simulink model "pitch_kalman_bias_sim"  (R2021b)
settings: Solver=VariableStepAuto  StartTime=0.0  StopTime=10.0  RelTol=1e-3
values from neighbouring files (symbols this model uses):
  A = [0 w_0(3) -w_0(2) 0 x_0(3) -x_0(2) ... (first row only)    [kalman_ex_5.m]    (also in pitch_kalman.m = 0; pitch_kalman_bias.m = [0 -1;0 0]; roll_kalman.m = 0; roll_kalman_bias.m = [0 -1;0 0])
  B = 1    [pitch_kalman.m]    (also in pitch_kalman_bias.m = [1;0]; roll_kalman.m; roll_kalman_bias.m = [1;0])
  bias = -0.3*ones(3,1)    [kalman_ex_5.m]    (also in pitch_kalman_bias.m = -0.3; roll_kalman_bias.m = -0.3)
  C = [eye(3) zeros(3,3)]    [kalman_ex_5.m]    (also in pitch_kalman.m = 1; pitch_kalman_bias.m = [1 0]; roll_kalman.m = 1; roll_kalman_bias.m = [1 0])
undefined symbols (not defined in the file or in its folder): L
settings Model: Creator=p28ma  LastModifiedBy=p28ma

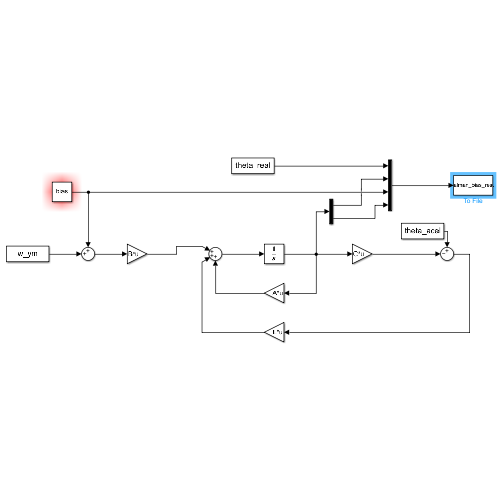
[thumbnail: Simulink's stored preview of the top-level diagram]
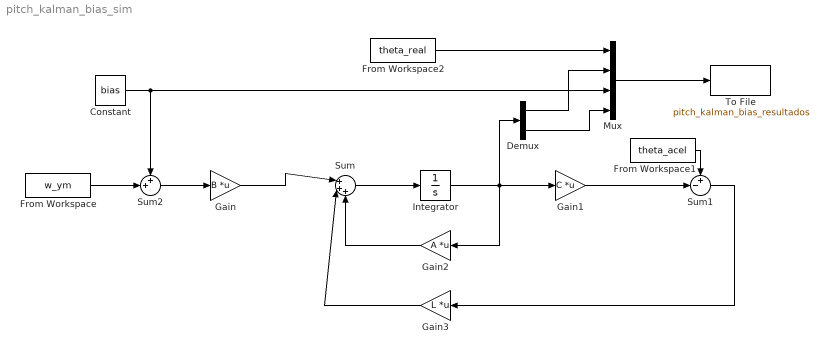
== system pitch_kalman_bias_sim ==
  Constant : Constant  Value=bias
  Demux : Demux  Outputs=2
  From Workspace : FromWorkspace  VariableName=w_ym  OutputAfterFinalValue=Setting to zero
  From Workspace1 : FromWorkspace  VariableName=theta_acel
  From Workspace2 : FromWorkspace  VariableName=theta_real
  Gain : Gain  Gain=B  Multiplication=Matrix(K*u)
  Gain1 : Gain  Gain=C  Multiplication=Matrix(K*u)
  Gain2 : Gain  Gain=A  Multiplication=Matrix(K*u)
  Gain3 : Gain  Gain=L  Multiplication=Matrix(K*u)
  Integrator : Integrator
  Mux : Mux
  Sum : Sum  Inputs=|+++
  Sum1 : Sum  Inputs=+-|
  Sum2 : Sum  Inputs=++|
  To File : ToFile  Filename=pitch_kalman_bias_resultados  MatrixName=pitch_kalman_bias_resultados  SaveFormat=Timeseries
  wires:
  Gain/1 -> Sum/1
  Sum/1 -> Integrator/1
  Integrator/1 -> Demux/1, Gain2/1, Gain1/1
  Gain2/1 -> Sum/3
  Sum1/1 -> Gain3/1
  Gain3/1 -> Sum/2
  Gain1/1 -> Sum1/2
  From Workspace1/1 -> Sum1/1
  Mux/1 -> To File/1
  From Workspace/1 -> Sum2/2
  Constant/1 -> Sum2/1, Mux/3
  Sum2/1 -> Gain/1
  From Workspace2/1 -> Mux/1
  Demux/1 -> Mux/2
  Demux/2 -> Mux/4
